simulink model "test_ibob_data_mux_10_1"  (Simulink 7.0)
settings: Solver=ode45  StartTime=0.0  StopTime=3000  RelTol=1e-3
libraries: xbsIndex_r4 x218, xbsReplacements_r4 x24, xps_library x3, xbsIndex_r3 x1
(part 1 of 2)
settings Model: Creator=Jason Manley  LastModifiedBy=Jason Manley
settings DebuggingCC: SaveWithParameterizedLinksMsg=none  SignalResolutionControl=TryResolveAllWithWarning  MultiTaskDSMMsg=warning  MultiTaskCondExecSysMsg=none  StrictBusMsg=None
settings RTWCC: IncludeERTFirstTime=on
settings GRTTargetCC: TargetFcnLib=ansi_tfl_tmw.mat

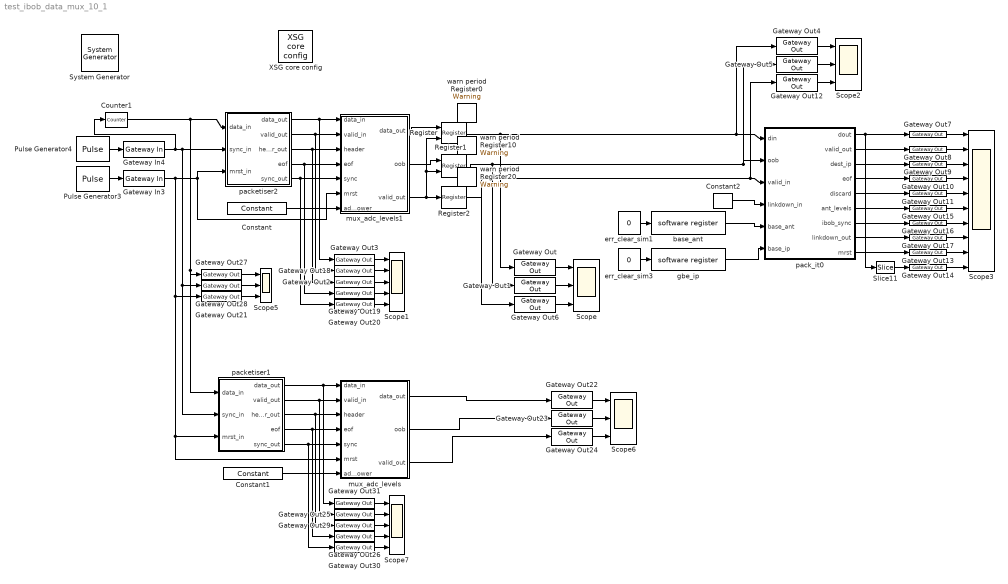
== system test_ibob_data_mux_10_1 ==
  " System Generator" : xbsIndex_r4/ System Generator  Tag=genX  SystemSampleTime=-1  xilinxfamily=Virtex2P  part=xc2vp50  speed=-7  package=ff1152  synthesis_tool=XST  clock_wrapper=Clock Enables  directory=./cn_i_128w_2k_x_rev3_astro_lib/sysgen  testbench=off  simulink_period=1  sysclk_period=5  dcm_input_clock_period=100  incr_netlist=off  trim_vbits=Everywhere in SubSystem  dbl_ovrd=According to Block Masks  core_generation=According to Block Masks  run_coregen=off  deprecated_control=off  eval_field=0  block_type=sysgen
      settings: block_version=10.1.3
  Constant : xbsIndex_r4/Constant  arith_type=Unsigned  const=(2^64) -1  n_bits=64  bin_pt=0  explicit_period=on  period=1  equ=P=C  opselect=C  inp2=PCIN>>17  opr=+  inp1=P  carry=CIN  dbl_ovrd=off  block_type=constant
  Constant1 : xbsIndex_r4/Constant  arith_type=Unsigned  const=(2^64) -1  n_bits=64  bin_pt=0  explicit_period=on  period=1  equ=P=C  opselect=C  inp2=PCIN>>17  opr=+  inp1=P  carry=CIN  dbl_ovrd=off  block_type=constant
  Constant2 : xbsIndex_r4/Constant  arith_type=Boolean  const=0  n_bits=1  bin_pt=0  explicit_period=on  period=1  equ=P=C  opselect=C  inp2=PCIN>>17  opr=+  inp1=P  carry=CIN  dbl_ovrd=off  block_type=constant
  Counter1 : xbsIndex_r3/Counter  cnt_type=Count Limited  n_bits=64  bin_pt=0  arith_type=Unsigned  start_count=0  cnt_to=Inf  cnt_by_val=1  operation=Up  explicit_period=off  period=1  load_pin=off  rst=on  en=off  dbl_ovrd=off  show_param=off  use_rpm=on  gen_core=off
      settings: xl_area=[0, 0, 0, 0, 0, 0, 0]
  Gateway In3 : xbsIndex_r4/Gateway In  arith_type=Boolean  n_bits=1  bin_pt=0  quantization=Truncate  overflow=Wrap  period=1  dbl_ovrd=off  timing_constraint=None  locs_specified=off  LOCs={}  block_type=gatewayin
      settings: infoedit="Gateway in block.  Converts inputs of type Simulink integer, double and fixed point to  Xilinx fixed point type.<P><P>Hardware notes:  In hardware these blocks become top level input ports."  xl_area=[0, 0, 0, 0, 0, 0, 0]  block_version=10.1.3
  Gateway In4 : xbsIndex_r4/Gateway In  arith_type=Boolean  n_bits=1  bin_pt=0  quantization=Truncate  overflow=Wrap  period=1  dbl_ovrd=off  timing_constraint=None  locs_specified=off  LOCs={}  block_type=gatewayin
      settings: infoedit="Gateway in block.  Converts inputs of type Simulink integer, double and fixed point to  Xilinx fixed point type.<P><P>Hardware notes:  In hardware these blocks become top level input ports."  xl_area=[0, 0, 0, 0, 0, 0, 0]  block_version=10.1.3
  Gateway Out{,1..31} (32 alike) : xbsIndex_r4/Gateway Out  hdl_port=on  timing_constraint=None  locs_specified=off  LOCs={}  block_type=gatewayout
      settings: infoedit="Gateway out block.  Converts Xilinx fixed point inputs into ouputs of type Simulink integer, double, or fixed point.<P><P>Hardware notes:  In hardware these blocks become top level output ports or are discarded, depending on how they are configured."  xl_area=[0, 0, 0, 0, 0, 0, 0]  block_version=10.1.3
  Pulse Generator3 : DiscretePulseGenerator  Period=40960  PhaseDelay=128
  Pulse Generator4 : DiscretePulseGenerator  Period=2048  PhaseDelay=150
  Register : xbsIndex_r4/Register  init=0  rst=off  en=on  dbl_ovrd=off  block_type=register
      settings: xl_area=[0, 0, 0, 0, 0, 0, 0]
  Register1 : xbsIndex_r4/Register  init=0  rst=off  en=on  dbl_ovrd=off  block_type=register
      settings: xl_area=[0, 0, 0, 0, 0, 0, 0]
  Register2 : xbsIndex_r4/Register  init=0  rst=off  en=off  dbl_ovrd=off  block_type=register
      settings: xl_area=[0, 0, 0, 0, 0, 0, 0]
  Scope{,2,5..6} (4 alike) : Scope  NumInputPorts=3
      Scope settings: YMin=-1.67772e+007~0~-5  YMax=4.5e+023~1~5
      Scope2 settings: YMin=0.95~-1~-1  YMax=1.05~1~1  SaveName=ScopeData5
      Scope5 settings: YMin=0~0~0  YMax=1800~1~1
      Scope6 settings: YMin=-1.67772e+007~0~-5  YMax=4.5e+023~1~5  SaveName=ScopeData10
  Scope1 : Scope  NumInputPorts=5
      settings: YMin=0~0~0~-5~-5  YMax=1.9e+014~1~1~5~5  SaveName=packetizer_out
  Scope3 : Scope  NumInputPorts=10
      settings: YMin=0~0~0~0~0~-5~-5~-5~-5~-5  YMax=1~5000~1~3~1~5~5~5~5~5  SaveName=ScopeData4
  Scope7 : Scope  NumInputPorts=5
      settings: YMin=0~0~0~-5~-5  YMax=1.9e+014~1~1~5~5  SaveName=packetizer_out1
  Slice11 : xbsIndex_r4/Slice  nbits=11  boolean_output=off  mode=Lower Bit Location + Width  bit1=0  base1=MSB of Input  bit0=16  base0=LSB of Input  dbl_ovrd=off  block_type=slice
      settings: infoedit="Extracts a given range of bits from each input sample and presents it at the output.  The output type is ordinarily unsigned with binary point at zero, but can be Boolean when the slice is one bit wide.<P><P>Hardware notes: In hardware this block costs nothing."  block_version=10.1.3
  XSG core config : xps_library/XSG core config  Tag=xps:xsg  SystemSampleTime=-1  hw_sys=iBOB  ibob_linux=off  clk_src=sys_clk  iBOB_clk_src=sys_clk  BEE2_ctrl_clk_src=sys_clk  BEE2_usr_clk_src=sys_clk  ROACH_clk_src=arb_clk  CORR_clk_src=sys_clk  gpio_clk_io_group=iBOB:sma  gpio_clk_bit_index=0  clk_rate=100  sample_period=1  synthesis_tool=XST  mpc_type=powerpc405
  base_ant : xps_library/software register  Tag=xps:sw_reg  SystemSampleTime=-1  io_dir=From Processor  arith_type=Unsigned  bitwidth=32  bin_pt=0  sample_period=1  gw_name=test_ibob_data_mux_base_ant_user_data_out
  err_clear_sim1 : Constant  Value=0  OutDataType=sfix(16)  OutScaling=2^0
  err_clear_sim3 : Constant  Value=0  OutDataType=sfix(16)  OutScaling=2^0
  gbe_ip : xps_library/software register  Tag=xps:sw_reg  SystemSampleTime=-1  io_dir=From Processor  arith_type=Unsigned  bitwidth=32  bin_pt=0  sample_period=1  gw_name=test_ibob_data_mux_gbe_ip_user_data_out
  mux_adc_levels : Subsystem  mask{wait_time=2000}
      mask prompts: wait_time "Attempt to insert antenna levels how many clocks after sync?"
  mux_adc_levels1 : Subsystem  mask{wait_time=2000}
      mask prompts: wait_time "Attempt to insert antenna levels how many clocks after sync?"
  pack_it0 : Subsystem  mask{payload_len=32, ant_bits=3, xeng_bits=3, skip_xeng_bits=1, skip_ant_bits=1}
      mask prompts: payload_len "Payload Length (in 64 bit words)"; ant_bits "Number of Antennas (2^?)"; xeng_bits "Number of X engines (2^?)"; skip_xeng_bits "X engines per IP address (2^?)"; skip_ant_bits "Antennas per XAUI link (2^?)"
      mask help: Packetizes data coming in over a XAUI interface. A packet consists of a 64 bit header (48 bits of "mcnt" and 16 bits of antenna), followed by 64 x "payload" bits of payload. "Mcnt" (master count) is a counter which keeps track of how many packets have been transmitted since the last "mrst".
      mask init:
      | packet_len = payload_len + 1;
      | packet_bits = ceil(log2(packet_len));
      | payload_bits = ceil(log2(payload_len));
  packetiser1 : Subsystem  mask{nwrd_bits=5, ant_bits=1}
      mask prompts: nwrd_bits "Payload length: (in 64bit words) (2^n)"; ant_bits "Number of antennas on this link (2^n)"
      mask help: Package 32 bit data into 64 bits and identify data as coming from antenna 0 or 1
  packetiser2 : Subsystem  mask{nwrd_bits=5, ant_bits=1}
      mask prompts: nwrd_bits "Payload length: (in 64bit words) (2^n)"; ant_bits "Number of antennas on this link (2^n)"
      mask help: Package 32 bit data into 64 bits and identify data as coming from antenna 0 or 1
  warn period Register0 : xbsReplacements_r4/Warning  SystemSampleTime=-1  period=1
  warn period Register10 : xbsReplacements_r4/Warning  SystemSampleTime=-1  period=1
  warn period Register20 : xbsReplacements_r4/Warning  SystemSampleTime=-1  period=1
  wires:
  Gateway Out/1 -> Scope/1
  Gateway Out1/1 -> Scope/2
  Gateway Out6/1 -> Scope/3
  err_clear_sim1/1 -> base_ant/1
  err_clear_sim3/1 -> gbe_ip/1
  gbe_ip/1 -> pack_it0/6(base_ip)
  base_ant/1 -> pack_it0/5(base_ant)
  Constant2/1 -> pack_it0/4(linkdown_in)
  Register/1 -> Gateway Out/1, Gateway Out4/1, pack_it0/1(din)
  mux_adc_levels1/2(oob) -> Register1/1
  mux_adc_levels1/3(valid_out) -> Register2/1, Register/2, Register1/2
  pack_it0/1(dout) -> Gateway Out7/1, Slice11/1
  Gateway Out7/1 -> Scope3/1
  Gateway Out8/1 -> Scope3/2
  Gateway Out9/1 -> Scope3/3
  Gateway Out10/1 -> Scope3/4
  Gateway Out11/1 -> Scope3/5
  packetiser2/1(data_out) -> Gateway Out3/1, mux_adc_levels1/1(data_in)
  packetiser2/2(valid_out) -> Gateway Out18/1, mux_adc_levels1/2(valid_in)
  packetiser2/4(eof) -> Gateway Out19/1, mux_adc_levels1/4(eof)
  packetiser2/5(sync_out) -> Gateway Out20/1, mux_adc_levels1/5(sync)
  Gateway Out3/1 -> Scope1/1
  Gateway Out18/1 -> Scope1/2
  Gateway Out2/1 -> Scope1/3
  Gateway Out19/1 -> Scope1/4
  Gateway Out20/1 -> Scope1/5
  Constant/1 -> mux_adc_levels1/7(adc_power)
  Counter1/1 -> packetiser2/1(data_in), Gateway Out27/1, packetiser1/1(data_in)
  Gateway Out27/1 -> Scope5/1
  Gateway Out28/1 -> Scope5/2
  Pulse Generator3/1 -> Gateway In3/1
  Pulse Generator4/1 -> Gateway In4/1
  Gateway In3/1 -> mux_adc_levels1/6(mrst), packetiser2/3(mrst_in), Gateway Out21/1, packetiser1/3(mrst_in), mux_adc_levels/6(mrst)
  Gateway In4/1 -> packetiser2/2(sync_in), Gateway Out28/1, packetiser1/2(sync_in), Counter1/1
  Gateway Out21/1 -> Scope5/3
  packetiser2/3(header_out) -> Gateway Out2/1, mux_adc_levels1/3(header)
  pack_it0/2(valid_out) -> Gateway Out8/1
  pack_it0/3(dest_ip) -> Gateway Out9/1
  pack_it0/4(eof) -> Gateway Out10/1
  pack_it0/5(discard) -> Gateway Out11/1
  Gateway Out4/1 -> Scope2/1
  Gateway Out5/1 -> Scope2/2
  Gateway Out12/1 -> Scope2/3
  mux_adc_levels1/1(data_out) -> Register/1
  Register1/1 -> Gateway Out1/1, Gateway Out5/1, pack_it0/2(oob)
  Register2/1 -> Gateway Out6/1, Gateway Out12/1, pack_it0/3(valid_in)
  pack_it0/6(ant_levels) -> Gateway Out15/1
  pack_it0/7(ibob_sync) -> Gateway Out16/1
  pack_it0/8(linkdown_out) -> Gateway Out17/1
  pack_it0/9(mrst) -> Gateway Out13/1
  packetiser1/1(data_out) -> mux_adc_levels/1(data_in), Gateway Out31/1
  packetiser1/2(valid_out) -> mux_adc_levels/2(valid_in), Gateway Out25/1
  packetiser1/3(header_out) -> mux_adc_levels/3(header), Gateway Out29/1
  packetiser1/4(eof) -> mux_adc_levels/4(eof), Gateway Out26/1
  packetiser1/5(sync_out) -> mux_adc_levels/5(sync), Gateway Out30/1
  Gateway Out22/1 -> Scope6/1
  Gateway Out23/1 -> Scope6/2
  Gateway Out24/1 -> Scope6/3
  mux_adc_levels/1(data_out) -> Gateway Out22/1
  mux_adc_levels/2(oob) -> Gateway Out23/1
  mux_adc_levels/3(valid_out) -> Gateway Out24/1
  Constant1/1 -> mux_adc_levels/7(adc_power)
  Gateway Out31/1 -> Scope7/1
  Gateway Out25/1 -> Scope7/2
  Gateway Out29/1 -> Scope7/3
  Gateway Out26/1 -> Scope7/4
  Gateway Out30/1 -> Scope7/5
  Gateway Out15/1 -> Scope3/6
  Gateway Out16/1 -> Scope3/7
  Gateway Out17/1 -> Scope3/8
  Gateway Out13/1 -> Scope3/9
  Gateway Out14/1 -> Scope3/10
  Slice11/1 -> Gateway Out14/1

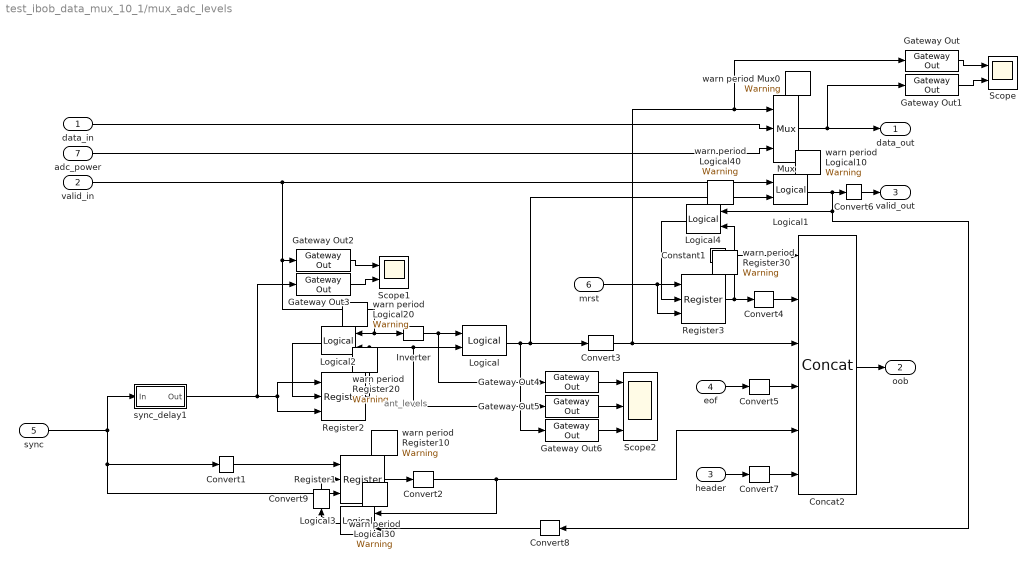
== system test_ibob_data_mux_10_1/mux_adc_levels ==
  note: ant_levels
  data_in : Inport  OutDataType=sfix(16)  OutScaling=2^0
  valid_in : Inport  Port=2  OutDataType=sfix(16)  OutScaling=2^0
  header : Inport  Port=3  OutDataType=sfix(16)  OutScaling=2^0
  eof : Inport  Port=4  OutDataType=sfix(16)  OutScaling=2^0
  sync : Inport  Port=5  OutDataType=sfix(16)  OutScaling=2^0
  mrst : Inport  Port=6  OutDataType=sfix(16)  OutScaling=2^0
  adc_power : Inport  Port=7  OutDataType=sfix(16)  OutScaling=2^0
  Concat2 : xbsIndex_r4/Concat  num_inputs=6  dbl_ovrd=off  block_type=concat
      settings: block_version=10.1.3
  Constant1 : xbsIndex_r4/Constant  arith_type=Unsigned  const=0  n_bits=3  bin_pt=0  explicit_period=on  period=1  equ=P=C  opselect=C  inp2=PCIN>>17  opr=+  inp1=P  carry=CIN  dbl_ovrd=off  block_type=constant
  Convert{1..5,7} (6 alike) : xbsIndex_r4/Convert  arith_type=Unsigned  n_bits=1  bin_pt=0  quantization=Truncate  overflow=Wrap  latency=0  dbl_ovrd=off  pipeline=off  block_type=convert
      settings: xl_area=[0, 0, 0, 0, 0, 0, 0]  block_version=10.1.3
  Convert6 : xbsIndex_r4/Convert  arith_type=Boolean  n_bits=1  bin_pt=0  quantization=Truncate  overflow=Wrap  latency=0  dbl_ovrd=off  pipeline=off  block_type=convert
      settings: xl_area=[0, 0, 0, 0, 0, 0, 0]  block_version=10.1.3
  Convert8 : xbsIndex_r4/Convert  Orientation=left  arith_type=Unsigned  n_bits=1  bin_pt=0  quantization=Truncate  overflow=Wrap  latency=0  dbl_ovrd=off  pipeline=off  block_type=convert
      settings: xl_area=[0, 0, 0, 0, 0, 0, 0]  block_version=10.1.3
  Convert9 : xbsIndex_r4/Convert  Orientation=up  arith_type=Boolean  n_bits=1  bin_pt=0  quantization=Truncate  overflow=Wrap  latency=0  dbl_ovrd=off  pipeline=off  block_type=convert
      settings: xl_area=[0, 0, 0, 0, 0, 0, 0]  block_version=10.1.3
  Gateway Out{,1..6} (7 alike) : xbsIndex_r4/Gateway Out  hdl_port=on  timing_constraint=None  locs_specified=off  LOCs={}  block_type=gatewayout
      settings: infoedit="Gateway out block.  Converts Xilinx fixed point inputs into ouputs of type Simulink integer, double, or fixed point.<P><P>Hardware notes:  In hardware these blocks become top level output ports or are discarded, depending on how they are configured."  xl_area=[0, 0, 0, 0, 0, 0, 0]  block_version=10.1.3
  Inverter : xbsIndex_r4/Inverter  en=off  latency=0  dbl_ovrd=off  block_type=inv
      settings: xl_area=[0, 0, 0, 0, 0, 0, 0]
  Logical : xbsIndex_r4/Logical  logical_function=AND  inputs=2  en=off  latency=0  precision=Full  arith_type=Unsigned  n_bits=8  bin_pt=2  align_bp=off  dbl_ovrd=off  block_type=logical
      settings: xl_area=[0, 0, 0, 0, 0, 0, 0]
  Logical1 : xbsIndex_r4/Logical  logical_function=OR  inputs=2  en=off  latency=0  precision=Full  arith_type=Unsigned  n_bits=8  bin_pt=2  align_bp=on  dbl_ovrd=off  block_type=logical
      settings: xl_area=[0, 0, 0, 0, 0, 0, 0]
  Logical2 : xbsIndex_r4/Logical  Orientation=left  logical_function=AND  inputs=2  en=off  latency=0  precision=Full  arith_type=Unsigned  n_bits=1  bin_pt=0  align_bp=off  dbl_ovrd=off  block_type=logical
      settings: xl_area=[0, 0, 0, 0, 0, 0, 0]
  Logical3 : xbsIndex_r4/Logical  Orientation=left  logical_function=AND  inputs=2  en=off  latency=0  precision=Full  arith_type=Unsigned  n_bits=1  bin_pt=0  align_bp=off  dbl_ovrd=off  block_type=logical
      settings: xl_area=[0, 0, 0, 0, 0, 0, 0]
  Logical4 : xbsIndex_r4/Logical  Orientation=left  logical_function=AND  inputs=2  en=off  latency=0  precision=Full  arith_type=Unsigned  n_bits=1  bin_pt=0  align_bp=off  dbl_ovrd=off  block_type=logical
      settings: xl_area=[0, 0, 0, 0, 0, 0, 0]
  Mux : xbsIndex_r4/Mux  inputs=2  en=off  latency=0  precision=Full  arith_type="Signed  (2's comp)"  n_bits=8  bin_pt=2  quantization=Truncate  overflow=Wrap  dbl_ovrd=off  block_type=mux
      settings: xl_area=[0, 0, 0, 0, 0, 0, 0]
  Register1 : xbsIndex_r4/Register  init=0  rst=on  en=on  dbl_ovrd=off  block_type=register
      settings: xl_area=[0, 0, 0, 0, 0, 0, 0]
  Register2 : xbsIndex_r4/Register  init=0  rst=on  en=on  dbl_ovrd=off  block_type=register
      settings: xl_area=[0, 0, 0, 0, 0, 0, 0]
  Register3 : xbsIndex_r4/Register  init=0  rst=on  en=on  dbl_ovrd=off  block_type=register
      settings: xl_area=[0, 0, 0, 0, 0, 0, 0]
  Scope : Scope  NumInputPorts=2
      settings: YMin=0~-1e+022  YMax=2~1.7e+023  SaveName=ScopeData3
  Scope1 : Scope  NumInputPorts=2
      settings: YMin=0~-1e+022  YMax=2~1.7e+023  SaveName=ScopeData2
  Scope2 : Scope  NumInputPorts=3
      settings: YMin=-1.67772e+007~0~-5  YMax=4.5e+023~1~5  SaveName=ScopeData11
  sync_delay1 : Subsystem  mask(sync_delay){DelayLen=wait_time}
      mask prompts: DelayLen "Delay Length:"
      mask help: Delay an infrequent boolean pulse by the specified number of clocks.
      mask init:
      | BitWidth = max(2, ceil(log2(DelayLen+1)));
      | UseCounter = 1;
      | if DelayLen == 0,
      | 	UseCounter = 0;
      | end
      mask Help: eval('xlWeb([getenv(''MLIB_ROOT''), ''\casper_library\doc\sync_delay_usage.html''])')
      mask Display: fprintf('Z^-%d', DelayLen)
  warn period Logical{10,20,30,40} (4 alike) : xbsReplacements_r4/Warning  SystemSampleTime=-1  period=1
  warn period Mux0 : xbsReplacements_r4/Warning  SystemSampleTime=-1  period=1
  warn period Register10 : xbsReplacements_r4/Warning  SystemSampleTime=-1  period=1
  warn period Register20 : xbsReplacements_r4/Warning  SystemSampleTime=-1  period=1
  warn period Register30 : xbsReplacements_r4/Warning  SystemSampleTime=-1  period=1
  data_out : Outport  OutDataType=sfix(16)  OutScaling=2^0
  oob : Outport  Port=2  OutDataType=sfix(16)  OutScaling=2^0
  valid_out : Outport  Port=3  OutDataType=sfix(16)  OutScaling=2^0
  wires:
  Concat2/1 -> oob/1
  sync/1 -> sync_delay1/1(In), Register1/3, Convert1/1
  Mux/1 -> data_out/1, Gateway Out1/1
  data_in/1 -> Mux/2
  adc_power/1 -> Mux/3
  Logical1/1 -> Logical4/1, Convert8/1, Convert6/1
  valid_in/1 -> Logical1/1, Gateway Out2/1, Logical2/1, Inverter/1
  Register2/1 -> Logical2/2, Gateway Out5/1, Logical/2
  sync_delay1/1(Out) -> Register2/1, Register2/3, Gateway Out3/1
  Gateway Out/1 -> Scope/1
  Gateway Out1/1 -> Scope/2
  Constant1/1 -> Concat2/1
  eof/1 -> Convert5/1
  header/1 -> Convert7/1
  Gateway Out2/1 -> Scope1/1
  Gateway Out3/1 -> Scope1/2
  Logical2/1 -> Register2/2
  Gateway Out4/1 -> Scope2/1
  Gateway Out5/1 -> Scope2/2
  Gateway Out6/1 -> Scope2/3
  Logical/1 -> Gateway Out6/1, Convert3/1, Logical1/2
  Convert3/1 -> Concat2/3, Mux/1, Gateway Out/1
  Inverter/1 -> Gateway Out4/1, Logical/1
  Register1/1 -> Convert2/1
  Register3/1 -> Logical4/2, Convert4/1
  mrst/1 -> Register3/1, Register3/3
  Logical3/1 -> Convert9/1
  Logical4/1 -> Register3/2
  Convert6/1 -> valid_out/1
  Convert4/1 -> Concat2/2
  Convert5/1 -> Concat2/4
  Convert7/1 -> Concat2/6
  Convert2/1 -> Concat2/5, Logical3/1
  Convert8/1 -> Logical3/2
  Convert9/1 -> Register1/2
  Convert1/1 -> Register1/1

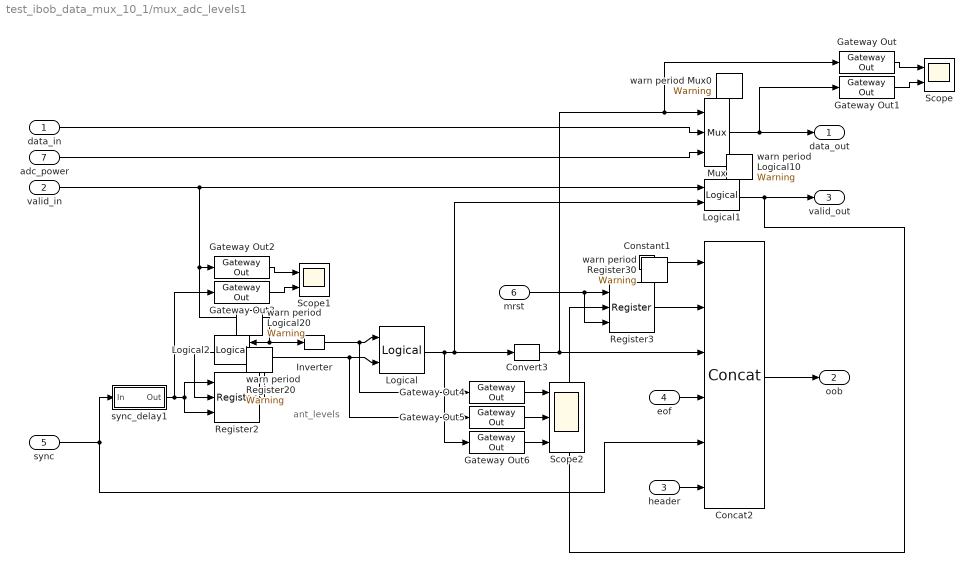
== system test_ibob_data_mux_10_1/mux_adc_levels1 ==
  note: ant_levels
  data_in : Inport  OutDataType=sfix(16)  OutScaling=2^0
  valid_in : Inport  Port=2  OutDataType=sfix(16)  OutScaling=2^0
  header : Inport  Port=3  OutDataType=sfix(16)  OutScaling=2^0
  eof : Inport  Port=4  OutDataType=sfix(16)  OutScaling=2^0
  sync : Inport  Port=5  OutDataType=sfix(16)  OutScaling=2^0
  mrst : Inport  Port=6  OutDataType=sfix(16)  OutScaling=2^0
  adc_power : Inport  Port=7  OutDataType=sfix(16)  OutScaling=2^0
  Concat2 : xbsIndex_r4/Concat  num_inputs=6  dbl_ovrd=off  block_type=concat
      settings: block_version=10.1.3
  Constant1 : xbsIndex_r4/Constant  arith_type=Unsigned  const=0  n_bits=3  bin_pt=0  explicit_period=on  period=1  equ=P=C  opselect=C  inp2=PCIN>>17  opr=+  inp1=P  carry=CIN  dbl_ovrd=off  block_type=constant
  Convert3 : xbsIndex_r4/Convert  arith_type=Unsigned  n_bits=1  bin_pt=0  quantization=Truncate  overflow=Wrap  latency=0  dbl_ovrd=off  pipeline=off  block_type=convert
      settings: xl_area=[0, 0, 0, 0, 0, 0, 0]  block_version=10.1.3
  Gateway Out{,1..6} (7 alike) : xbsIndex_r4/Gateway Out  hdl_port=on  timing_constraint=None  locs_specified=off  LOCs={}  block_type=gatewayout
      settings: infoedit="Gateway out block.  Converts Xilinx fixed point inputs into ouputs of type Simulink integer, double, or fixed point.<P><P>Hardware notes:  In hardware these blocks become top level output ports or are discarded, depending on how they are configured."  xl_area=[0, 0, 0, 0, 0, 0, 0]  block_version=10.1.3
  Inverter : xbsIndex_r4/Inverter  en=off  latency=0  dbl_ovrd=off  block_type=inv
      settings: xl_area=[0, 0, 0, 0, 0, 0, 0]
  Logical : xbsIndex_r4/Logical  logical_function=AND  inputs=2  en=off  latency=0  precision=Full  arith_type=Unsigned  n_bits=8  bin_pt=2  align_bp=off  dbl_ovrd=off  block_type=logical
      settings: xl_area=[0, 0, 0, 0, 0, 0, 0]
  Logical1 : xbsIndex_r4/Logical  logical_function=OR  inputs=2  en=off  latency=0  precision=Full  arith_type=Unsigned  n_bits=8  bin_pt=2  align_bp=on  dbl_ovrd=off  block_type=logical
      settings: xl_area=[0, 0, 0, 0, 0, 0, 0]
  Logical2 : xbsIndex_r4/Logical  Orientation=left  logical_function=AND  inputs=2  en=off  latency=0  precision=Full  arith_type=Unsigned  n_bits=1  bin_pt=0  align_bp=off  dbl_ovrd=off  block_type=logical
      settings: xl_area=[0, 0, 0, 0, 0, 0, 0]
  Mux : xbsIndex_r4/Mux  inputs=2  en=off  latency=0  precision=Full  arith_type="Signed  (2's comp)"  n_bits=8  bin_pt=2  quantization=Truncate  overflow=Wrap  dbl_ovrd=off  block_type=mux
      settings: xl_area=[0, 0, 0, 0, 0, 0, 0]
  Register2 : xbsIndex_r4/Register  init=0  rst=on  en=on  dbl_ovrd=off  block_type=register
      settings: xl_area=[0, 0, 0, 0, 0, 0, 0]
  Register3 : xbsIndex_r4/Register  init=0  rst=on  en=on  dbl_ovrd=off  block_type=register
      settings: xl_area=[0, 0, 0, 0, 0, 0, 0]
  Scope : Scope  NumInputPorts=2
      settings: YMin=0~-1e+022  YMax=2~1.7e+023  SaveName=ScopeData3
  Scope1 : Scope  NumInputPorts=2
      settings: YMin=0~-1e+022  YMax=2~1.7e+023  SaveName=ScopeData2
  Scope2 : Scope  NumInputPorts=3
      settings: YMin=-1.67772e+007~0~-5  YMax=4.5e+023~1~5  SaveName=ScopeData11
  sync_delay1 : Subsystem  mask(sync_delay){DelayLen=wait_time}
      mask prompts: DelayLen "Delay Length:"
      mask help: Delay an infrequent boolean pulse by the specified number of clocks.
      mask init:
      | BitWidth = max(2, ceil(log2(DelayLen+1)));
      | UseCounter = 1;
      | if DelayLen == 0,
      | 	UseCounter = 0;
      | end
      mask Help: eval('xlWeb([getenv(''MLIB_ROOT''), ''\casper_library\doc\sync_delay_usage.html''])')
      mask Display: fprintf('Z^-%d', DelayLen)
  warn period Logical10 : xbsReplacements_r4/Warning  SystemSampleTime=-1  period=1
  warn period Logical20 : xbsReplacements_r4/Warning  SystemSampleTime=-1  period=1
  warn period Mux0 : xbsReplacements_r4/Warning  SystemSampleTime=-1  period=1
  warn period Register20 : xbsReplacements_r4/Warning  SystemSampleTime=-1  period=1
  warn period Register30 : xbsReplacements_r4/Warning  SystemSampleTime=-1  period=1
  data_out : Outport  OutDataType=sfix(16)  OutScaling=2^0
  oob : Outport  Port=2  OutDataType=sfix(16)  OutScaling=2^0
  valid_out : Outport  Port=3  OutDataType=sfix(16)  OutScaling=2^0
  wires:
  Concat2/1 -> oob/1
  sync/1 -> sync_delay1/1(In), Concat2/5
  Mux/1 -> data_out/1, Gateway Out1/1
  data_in/1 -> Mux/2
  adc_power/1 -> Mux/3
  Logical1/1 -> valid_out/1, Register3/2
  valid_in/1 -> Logical1/1, Gateway Out2/1, Logical2/1, Inverter/1
  Register2/1 -> Logical2/2, Gateway Out5/1, Logical/2
  sync_delay1/1(Out) -> Register2/1, Register2/3, Gateway Out3/1
  Gateway Out/1 -> Scope/1
  Gateway Out1/1 -> Scope/2
  Constant1/1 -> Concat2/1
  eof/1 -> Concat2/4
  header/1 -> Concat2/6
  Gateway Out2/1 -> Scope1/1
  Gateway Out3/1 -> Scope1/2
  Logical2/1 -> Register2/2
  Gateway Out4/1 -> Scope2/1
  Gateway Out5/1 -> Scope2/2
  Gateway Out6/1 -> Scope2/3
  Logical/1 -> Gateway Out6/1, Convert3/1, Logical1/2
  Convert3/1 -> Concat2/3, Mux/1, Gateway Out/1
  Inverter/1 -> Gateway Out4/1, Logical/1
  Register3/1 -> Concat2/2
  mrst/1 -> Register3/1, Register3/3

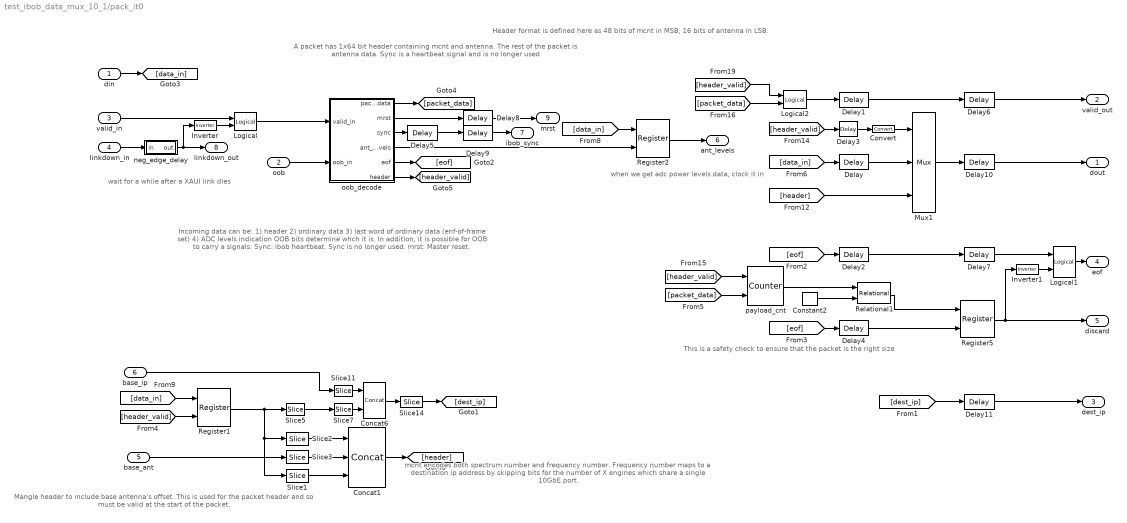
== system test_ibob_data_mux_10_1/pack_it0 ==
  note: mcnt encodes both spectrum number
      | and frequency number.  Frequency number
      | maps to a destination ip address by skipping
      | bits for the number of X engines which
      | share a single 10GbE port.
  note: A packet has 1x64 bit header
      | containing mcnt and antenna.
      | The rest of the packet is antenna data.
      |
      | Sync is a heartbeat signal and is no longer used
  note: This is a safety check to ensure that the packet is the right size
  note: wait for a while after a XAUI link dies
  note: Incoming data can be:
      | 1) header
      | 2) ordinary data
      | 3) last word of ordinary data (enf-of-frame set)
      | 4) ADC levels indication
      |  OOB bits determine whch it is.
      | In addition, it is possible for OOB to carry a signals:
      | Sync: ibob heartbeat. Sync is no longer used.
      | mrst: Master reset.
  note: when we get adc power levels
      | data, clock it in
  note: Mangle header to include base antenna's offset.
      | This is used for the packet header and so must be valid at the start of the packet.
  note: Header format is defined here
      | as 48 bits of mcnt in MSB, 16 bits of
      | antenna in LSB.
  din : Inport  OutDataType=sfix(16)  OutScaling=2^0
  oob : Inport  Port=2  OutDataType=sfix(16)  OutScaling=2^0
  valid_in : Inport  Port=3  OutDataType=sfix(16)  OutScaling=2^0
  linkdown_in : Inport  Port=4  OutDataType=sfix(16)  OutScaling=2^0
  base_ant : Inport  Port=5  OutDataType=sfix(16)  OutScaling=2^0
  base_ip : Inport  Port=6  OutDataType=sfix(16)  OutScaling=2^0
  Concat1 : xbsIndex_r4/Concat  num_inputs=3  dbl_ovrd=off  block_type=concat
      settings: block_version=10.1.3
  Concat6 : xbsIndex_r4/Concat  num_inputs=2  dbl_ovrd=off  block_type=concat
      settings: block_version=10.1.3
  Constant2 : xbsIndex_r4/Constant  arith_type=Unsigned  const=packet_len-1  n_bits=packet_bits+1  bin_pt=0  explicit_period=on  period=1  equ=P=C  opselect=C  inp2=PCIN>>17  opr=+  inp1=P  carry=CIN  dbl_ovrd=off  block_type=constant
  Convert : xbsIndex_r4/Convert  arith_type=Unsigned  n_bits=1  bin_pt=0  quantization=Truncate  overflow=Wrap  latency=0  dbl_ovrd=off  pipeline=off  block_type=convert
      settings: xl_area=[0, 0, 0, 0, 0, 0, 0]  block_version=10.1.3
  Delay{,1..11} (12 alike) : xbsIndex_r4/Delay  en=off  latency=1  dbl_ovrd=off  reg_retiming=on  block_type=delay
      settings: xl_area=[0, 0, 0, 0, 0, 0, 0]
  Inverter : xbsIndex_r4/Inverter  en=off  latency=0  dbl_ovrd=off  block_type=inv
      settings: xl_area=[0, 0, 0, 0, 0, 0, 0]
  Inverter1 : xbsIndex_r4/Inverter  en=off  latency=0  dbl_ovrd=off  block_type=inv
      settings: xl_area=[0, 0, 0, 0, 0, 0, 0]
  Logical : xbsIndex_r4/Logical  logical_function=AND  inputs=2  en=off  latency=0  precision=Full  arith_type=Unsigned  n_bits=8  bin_pt=2  align_bp=on  dbl_ovrd=off  block_type=logical
      settings: xl_area=[0, 0, 0, 0, 0, 0, 0]
  Logical1 : xbsIndex_r4/Logical  logical_function=AND  inputs=2  en=off  latency=0  precision=Full  arith_type=Unsigned  n_bits=8  bin_pt=2  align_bp=on  dbl_ovrd=off  block_type=logical
      settings: xl_area=[0, 0, 0, 0, 0, 0, 0]
  Logical2 : xbsIndex_r4/Logical  logical_function=OR  inputs=2  en=off  latency=0  precision=Full  arith_type=Unsigned  n_bits=8  bin_pt=2  align_bp=on  dbl_ovrd=off  block_type=logical
      settings: xl_area=[0, 0, 0, 0, 0, 0, 0]
  Mux1 : xbsIndex_r4/Mux  inputs=2  en=off  latency=0  precision=Full  arith_type="Signed  (2's comp)"  n_bits=8  bin_pt=2  quantization=Truncate  overflow=Wrap  dbl_ovrd=off  block_type=mux
      settings: xl_area=[0, 0, 0, 0, 0, 0, 0]
  Register1 : xbsIndex_r4/Register  init=0  rst=off  en=on  dbl_ovrd=off  block_type=register
      settings: xl_area=[0, 0, 0, 0, 0, 0, 0]
  Register2 : xbsIndex_r4/Register  init=0  rst=off  en=on  dbl_ovrd=off  block_type=register
      settings: xl_area=[0, 0, 0, 0, 0, 0, 0]
  Register5 : xbsIndex_r4/Register  init=0  rst=off  en=on  dbl_ovrd=off  block_type=register
      settings: xl_area=[0, 0, 0, 0, 0, 0, 0]
  Relational1 : xbsIndex_r4/Relational  mode=a!=b  en=off  latency=0  dbl_ovrd=off  block_type=relational
      settings: xl_area=[0, 0, 0, 0, 0, 0, 0]  block_version=10.1.3
  Slice1 : xbsIndex_r4/Slice  nbits=skip_ant_bits  boolean_output=off  mode=Lower Bit Location + Width  bit1=0  base1=LSB of Input  bit0=0  base0=LSB of Input  dbl_ovrd=off  block_type=slice
      settings: infoedit="Extracts a given range of bits from each input sample and presents it at the output.  The output type is ordinarily unsigned with binary point at zero, but can be Boolean when the slice is one bit wide.<P><P>Hardware notes: In hardware this block costs nothing."  block_version=10.1.3
  Slice11 : xbsIndex_r4/Slice  nbits=32 - (xeng_bits - skip_xeng_bits)  boolean_output=off  mode=Upper Bit Location + Width  bit1=0  base1=MSB of Input  bit0=0  base0=LSB of Input  dbl_ovrd=off  block_type=slice
      settings: infoedit="Extracts a given range of bits from each input sample and presents it at the output.  The output type is ordinarily unsigned with binary point at zero, but can be Boolean when the slice is one bit wide.<P><P>Hardware notes: In hardware this block costs nothing."  block_version=10.1.3
  Slice14 : xbsIndex_r4/Slice  nbits=32  boolean_output=off  mode=Upper Bit Location + Width  bit1=0  base1=MSB of Input  bit0=0  base0=LSB of Input  dbl_ovrd=off  block_type=slice
      settings: infoedit="Extracts a given range of bits from each input sample and presents it at the output.  The output type is ordinarily unsigned with binary point at zero, but can be Boolean when the slice is one bit wide.<P><P>Hardware notes: In hardware this block costs nothing."  block_version=10.1.3
  Slice2 : xbsIndex_r4/Slice  nbits=48  boolean_output=off  mode=Lower Bit Location + Width  bit1=16  base1=MSB of Input  bit0=16  base0=LSB of Input  dbl_ovrd=off  block_type=slice
      settings: infoedit="Extracts a given range of bits from each input sample and presents it at the output.  The output type is ordinarily unsigned with binary point at zero, but can be Boolean when the slice is one bit wide.<P><P>Hardware notes: In hardware this block costs nothing."  block_version=10.1.3
  Slice3 : xbsIndex_r4/Slice  nbits=16-skip_ant_bits  boolean_output=off  mode=Lower Bit Location + Width  bit1=0  base1=LSB of Input  bit0=skip_ant_bits  base0=LSB of Input  dbl_ovrd=off  block_type=slice
      settings: infoedit="Extracts a given range of bits from each input sample and presents it at the output.  The output type is ordinarily unsigned with binary point at zero, but can be Boolean when the slice is one bit wide.<P><P>Hardware notes: In hardware this block costs nothing."  block_version=10.1.3
  Slice5 : xbsIndex_r4/Slice  nbits=xeng_bits - skip_xeng_bits  boolean_output=off  mode=Lower Bit Location + Width  bit1=0  base1=MSB of Input  bit0=16 + skip_xeng_bits  base0=LSB of Input  dbl_ovrd=off  block_type=slice
      settings: infoedit="Extracts a given range of bits from each input sample and presents it at the output.  The output type is ordinarily unsigned with binary point at zero, but can be Boolean when the slice is one bit wide.<P><P>Hardware notes: In hardware this block costs nothing."  block_version=10.1.3
  Slice7 : xbsIndex_r4/Slice  nbits=xeng_bits - skip_xeng_bits  boolean_output=off  mode=Lower Bit Location + Width  bit1=0  base1=MSB of Input  bit0=0  base0=LSB of Input  dbl_ovrd=off  block_type=slice
      settings: infoedit="Extracts a given range of bits from each input sample and presents it at the output.  The output type is ordinarily unsigned with binary point at zero, but can be Boolean when the slice is one bit wide.<P><P>Hardware notes: In hardware this block costs nothing."  block_version=10.1.3
  neg_edge_delay : Subsystem  AncestorBlock=casper_library/Misc/pulse_ext  mask(pulse_ext){pulse_len=5}
      mask prompts: pulse_len "Length of Pulse"
      mask help:
      | Extends a boolean signal to be high for the specified number of clocks after
      | the last high input.
      mask init:
      | bits = ceil(log2(pulse_len+1));
      mask Help: eval('xlWeb([getenv(''MLIB_ROOT''), ''\casper_library\doc\pulse_ext_usage.html''])')
  oob_decode : Subsystem
  payload_cnt : xbsIndex_r4/Counter  cnt_type=Free Running  cnt_to=packet_len - 1  operation=Up  start_count=0  cnt_by_val=1  arith_type=Unsigned  n_bits=packet_bits+1  bin_pt=0  load_pin=off  rst=on  en=on  explicit_period=off  period=1  dbl_ovrd=off  use_behavioral_HDL=off  use_rpm=on  implementation=Fabric  block_type=counter
      settings: xl_area=[0, 0, 0, 0, 0, 0, 0]
  dout : Outport  OutDataType=sfix(16)  OutScaling=2^0
  valid_out : Outport  Port=2  OutDataType=sfix(16)  OutScaling=2^0
  dest_ip : Outport  Port=3  OutDataType=sfix(16)  OutScaling=2^0
  eof : Outport  Port=4  OutDataType=sfix(16)  OutScaling=2^0
  discard : Outport  Port=5  OutDataType=sfix(16)  OutScaling=2^0
  ant_levels : Outport  Port=6  OutDataType=sfix(16)  OutScaling=2^0
  ibob_sync : Outport  Port=7  OutDataType=sfix(16)  OutScaling=2^0
  linkdown_out : Outport  Port=8  OutDataType=sfix(16)  OutScaling=2^0
  mrst : Outport  Port=9  OutDataType=sfix(16)  OutScaling=2^0
  wires:
  Mux1/1 -> Delay10/1
  payload_cnt/1 -> Relational1/1
  Constant2/1 -> Relational1/2
  [packet_data] -> payload_cnt/2
  Inverter/1 -> Logical/2
  neg_edge_delay/1(out) -> linkdown_out/1, Inverter/1
  valid_in/1 -> Logical/1
  Logical/1 -> oob_decode/1(valid_in)
  linkdown_in/1 -> neg_edge_delay/1(in)
  oob/1 -> oob_decode/2(oob_in)
  Register2/1 -> ant_levels/1
  din/1 -> [data_in]
  [data_in] -> Register2/1
  [header_valid] -> payload_cnt/1
  oob_decode/2(mrst) -> Delay8/1
  oob_decode/4(ant_levels) -> Register2/2
  oob_decode/3(sync) -> Delay5/1
  oob_decode/1(packet_data) -> [packet_data]
  Relational1/1 -> Register5/1
  Register5/1 -> discard/1, Inverter1/1
  oob_decode/6(header) -> [header_valid]
  Delay/1 -> Mux1/2
  [header_valid] -> Delay3/1
  base_ip/1 -> Slice11/1
  Slice11/1 -> Concat6/1
  Slice7/1 -> Concat6/2
  Concat6/1 -> Slice14/1
  [header_valid] -> Register1/2
  [data_in] -> Register1/1
  Slice2/1 -> Concat1/1
  Register1/1 -> Slice2/1, Slice1/1, Slice5/1
  Concat1/1 -> [header]
  Slice1/1 -> Concat1/3
  Slice3/1 -> Concat1/2
  base_ant/1 -> Slice3/1
  [header] -> Mux1/3
  Logical2/1 -> Delay1/1
  Delay1/1 -> Delay6/1
  Delay2/1 -> Delay7/1
  Convert/1 -> Mux1/1
  Delay3/1 -> Convert/1
  [data_in] -> Delay/1
  [packet_data] -> Logical2/2
  [header_valid] -> Logical2/1
  Delay5/1 -> Delay9/1
  Delay4/1 -> Register5/2
  Delay6/1 -> valid_out/1
  Delay8/1 -> mrst/1
  Delay9/1 -> ibob_sync/1
  Inverter1/1 -> Logical1/2
  Logical1/1 -> eof/1
  Delay7/1 -> Logical1/1
  Delay10/1 -> dout/1
  Slice5/1 -> Slice7/1
  Delay11/1 -> dest_ip/1
  Slice14/1 -> [dest_ip]
  [dest_ip] -> Delay11/1
  oob_decode/5(eof) -> [eof]
  [eof] -> Delay2/1
  [eof] -> Delay4/1

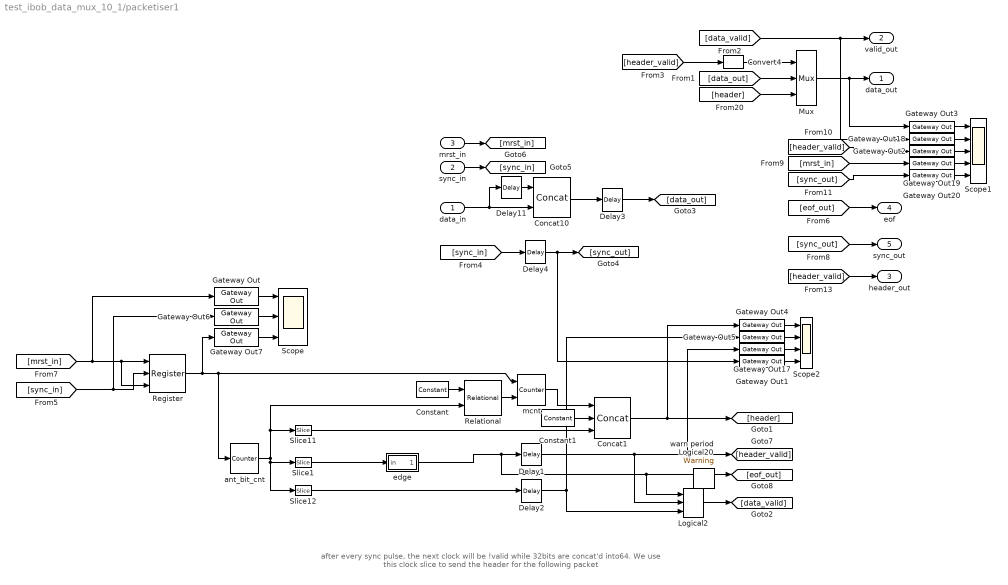
== system test_ibob_data_mux_10_1/packetiser1 ==
  note: after every sync pulse,
      | the next clock will be !valid while 32bits are concat'd into64.
      | We use this clock slice to send the header for the following packet
  data_in : Inport  OutDataType=sfix(16)  OutScaling=2^0
  sync_in : Inport  Port=2  OutDataType=sfix(16)  OutScaling=2^0
  mrst_in : Inport  Port=3  OutDataType=sfix(16)  OutScaling=2^0
  Concat1 : xbsIndex_r4/Concat  num_inputs=3  dbl_ovrd=off  block_type=concat
      settings: block_version=10.1.3
  Concat10 : xbsIndex_r4/Concat  num_inputs=2  dbl_ovrd=off  block_type=concat
      settings: block_version=10.1.3
  Constant : xbsIndex_r4/Constant  arith_type=Unsigned  const=0  n_bits=nwrd_bits+ant_bits+1  bin_pt=0  explicit_period=on  period=1  equ=P=C  opselect=C  inp2=PCIN>>17  opr=+  inp1=P  carry=CIN  dbl_ovrd=off  block_type=constant
  Constant1 : xbsIndex_r4/Constant  arith_type=Unsigned  const=0  n_bits=16-ant_bits  bin_pt=0  explicit_period=on  period=1  equ=P=C  opselect=C  inp2=PCIN>>17  opr=+  inp1=P  carry=CIN  dbl_ovrd=off  block_type=constant
  Convert4 : xbsIndex_r4/Convert  arith_type=Unsigned  n_bits=1  bin_pt=0  quantization=Truncate  overflow=Wrap  latency=0  dbl_ovrd=off  pipeline=off  block_type=convert
      settings: xl_area=[0, 0, 0, 0, 0, 0, 0]  block_version=10.1.3
  Delay{1,3..4,11} (4 alike) : xbsIndex_r4/Delay  en=off  latency=1  dbl_ovrd=off  reg_retiming=on  block_type=delay
      settings: xl_area=[0, 0, 0, 0, 0, 0, 0]
  Delay2 : xbsIndex_r4/Delay  en=off  latency=1  dbl_ovrd=off  reg_retiming=off  block_type=delay
      settings: xl_area=[0, 0, 0, 0, 0, 0, 0]
  Gateway Out{,1..7,17..20} (12 alike) : xbsIndex_r4/Gateway Out  hdl_port=on  timing_constraint=None  locs_specified=off  LOCs={}  block_type=gatewayout
      settings: infoedit="Gateway out block.  Converts Xilinx fixed point inputs into ouputs of type Simulink integer, double, or fixed point.<P><P>Hardware notes:  In hardware these blocks become top level output ports or are discarded, depending on how they are configured."  xl_area=[0, 0, 0, 0, 0, 0, 0]  block_version=10.1.3
  Logical2 : xbsIndex_r4/Logical  logical_function=OR  inputs=3  en=off  latency=0  precision=Full  arith_type=Unsigned  n_bits=1  bin_pt=0  align_bp=on  dbl_ovrd=off  block_type=logical
      settings: xl_area=[0, 0, 0, 0, 0, 0, 0]
  Mux : xbsIndex_r4/Mux  inputs=2  en=off  latency=0  precision=Full  arith_type="Signed  (2's comp)"  n_bits=8  bin_pt=2  quantization=Truncate  overflow=Wrap  dbl_ovrd=off  block_type=mux
      settings: xl_area=[0, 0, 0, 0, 0, 0, 0]
  Register : xbsIndex_r4/Register  init=0  rst=on  en=on  dbl_ovrd=off  block_type=register
      settings: xl_area=[0, 0, 0, 0, 0, 0, 0]
  Relational : xbsIndex_r4/Relational  mode=a=b  en=off  latency=0  dbl_ovrd=off  block_type=relational
      settings: xl_area=[0, 0, 0, 0, 0, 0, 0]  block_version=10.1.3
  Scope : Scope  NumInputPorts=3
      settings: YMin=-16777200~0~-5  YMax=4.5e+023~1~5  SaveName=ScopeData8
  Scope1 : Scope  NumInputPorts=5
      settings: YMin=0~0~0~-1~-1  YMax=4e+013~1~1~1~1  SaveName=ScopeData6
  Scope2 : Scope  NumInputPorts=4
      settings: YMin=0~0~0~-5  YMax=6.5e+006~1~1~5  SaveName=ScopeData7
  Slice1 : xbsIndex_r4/Slice  nbits=1  boolean_output=on  mode=Lower Bit Location + Width  bit1=0  base1=MSB of Input  bit0=nwrd_bits+1  base0=LSB of Input  dbl_ovrd=off  block_type=slice
      settings: infoedit="Extracts a given range of bits from each input sample and presents it at the output.  The output type is ordinarily unsigned with binary point at zero, but can be Boolean when the slice is one bit wide.<P><P>Hardware notes: In hardware this block costs nothing."  block_version=10.1.3
  Slice11 : xbsIndex_r4/Slice  nbits=ant_bits  boolean_output=on  mode=Lower Bit Location + Width  bit1=0  base1=MSB of Input  bit0=nwrd_bits+1  base0=LSB of Input  dbl_ovrd=off  block_type=slice
      settings: infoedit="Extracts a given range of bits from each input sample and presents it at the output.  The output type is ordinarily unsigned with binary point at zero, but can be Boolean when the slice is one bit wide.<P><P>Hardware notes: In hardware this block costs nothing."  block_version=10.1.3
  Slice12 : xbsIndex_r4/Slice  nbits=1  boolean_output=on  mode=Lower Bit Location + Width  bit1=0  base1=MSB of Input  bit0=0  base0=LSB of Input  dbl_ovrd=off  block_type=slice
      settings: infoedit="Extracts a given range of bits from each input sample and presents it at the output.  The output type is ordinarily unsigned with binary point at zero, but can be Boolean when the slice is one bit wide.<P><P>Hardware notes: In hardware this block costs nothing."  block_version=10.1.3
  ant_bit_cnt : xbsIndex_r4/Counter  cnt_type=Free Running  cnt_to=Inf  operation=Up  start_count=0  cnt_by_val=1  arith_type=Unsigned  n_bits=nwrd_bits+ant_bits+1  bin_pt=0  load_pin=off  rst=on  en=off  explicit_period=on  period=1  dbl_ovrd=off  use_behavioral_HDL=off  use_rpm=on  implementation=Fabric  block_type=counter
      settings: xl_area=[0, 0, 0, 0, 0, 0, 0]
  edge : Subsystem
      mask Type: edge
      mask Description: Outputs true if a boolean input signal is not equal to its value last clock.
      mask Help: eval('xlWeb([getenv(''MLIB_ROOT''), ''\casper_library\doc\edge_usage.html''])')
  mcnt : xbsIndex_r4/Counter  cnt_type=Free Running  cnt_to=Inf  operation=Up  start_count=0  cnt_by_val=1  arith_type=Unsigned  n_bits=48  bin_pt=0  load_pin=off  rst=on  en=on  explicit_period=off  period=1  dbl_ovrd=off  use_behavioral_HDL=off  use_rpm=on  implementation=Fabric  block_type=counter
      settings: xl_area=[0, 0, 0, 0, 0, 0, 0]
  warn period Logical20 : xbsReplacements_r4/Warning  SystemSampleTime=-1  period=1
  data_out : Outport  OutDataType=sfix(16)  OutScaling=2^0
  valid_out : Outport  Port=2  OutDataType=sfix(16)  OutScaling=2^0
  header_out : Outport  Port=3  OutDataType=sfix(16)  OutScaling=2^0
  eof : Outport  Port=4  OutDataType=sfix(16)  OutScaling=2^0
  sync_out : Outport  Port=5  OutDataType=sfix(16)  OutScaling=2^0
  wires:
  ant_bit_cnt/1 -> Slice11/1, Relational/2, Slice12/1, Slice1/1
  data_in/1 -> Delay11/1, Concat10/2
  Constant/1 -> Relational/1
  Relational/1 -> mcnt/2
  Slice1/1 -> edge/1(in)
  mcnt/1 -> Concat1/1
  Constant1/1 -> Concat1/2
  Slice11/1 -> Concat1/3
  Convert4/1 -> Mux/1
  Mux/1 -> data_out/1, Gateway Out3/1
  Concat1/1 -> [header], Gateway Out4/1
  [header] -> Mux/3
  [data_out] -> Mux/2
  Slice12/1 -> Delay2/1
  [data_valid] -> valid_out/1, Gateway Out18/1
  [header_valid] -> Convert4/1
  sync_in/1 -> [sync_in]
  mrst_in/1 -> [mrst_in]
  Register/1 -> ant_bit_cnt/1, mcnt/1, Gateway Out7/1
  [eof_out] -> eof/1
  [sync_out] -> sync_out/1
  Gateway Out3/1 -> Scope1/1
  Gateway Out18/1 -> Scope1/2
  Gateway Out2/1 -> Scope1/3
  Gateway Out19/1 -> Scope1/4
  Gateway Out20/1 -> Scope1/5
  [header_valid] -> Gateway Out2/1
  [mrst_in] -> Gateway Out19/1
  [sync_out] -> Gateway Out20/1
  Gateway Out4/1 -> Scope2/1
  Gateway Out5/1 -> Scope2/2
  Gateway Out17/1 -> Scope2/3
  [sync_in] -> Delay4/1
  edge/1(out) -> Delay1/1, [eof_out], Logical2/1
  Gateway Out1/1 -> Scope2/4
  Delay1/1 -> [header_valid], Gateway Out17/1, Logical2/2
  Delay2/1 -> Gateway Out5/1, Logical2/3
  Delay4/1 -> [sync_out], Gateway Out1/1
  [mrst_in] -> Gateway Out/1, Register/1, Register/3
  [sync_in] -> Register/2, Gateway Out6/1
  Gateway Out/1 -> Scope/1
  Gateway Out6/1 -> Scope/2
  Gateway Out7/1 -> Scope/3
  [header_valid] -> header_out/1
  Logical2/1 -> [data_valid]
  Delay11/1 -> Concat10/1
  Concat10/1 -> Delay3/1
  Delay3/1 -> [data_out]
